simulink model "C_rho"  (R2020a)
settings: Solver=VariableStepAuto  StartTime=0.0  StopTime=10.0  RelTol=1e-3
settings Model: Creator=Willie  LastModifiedBy=Willie

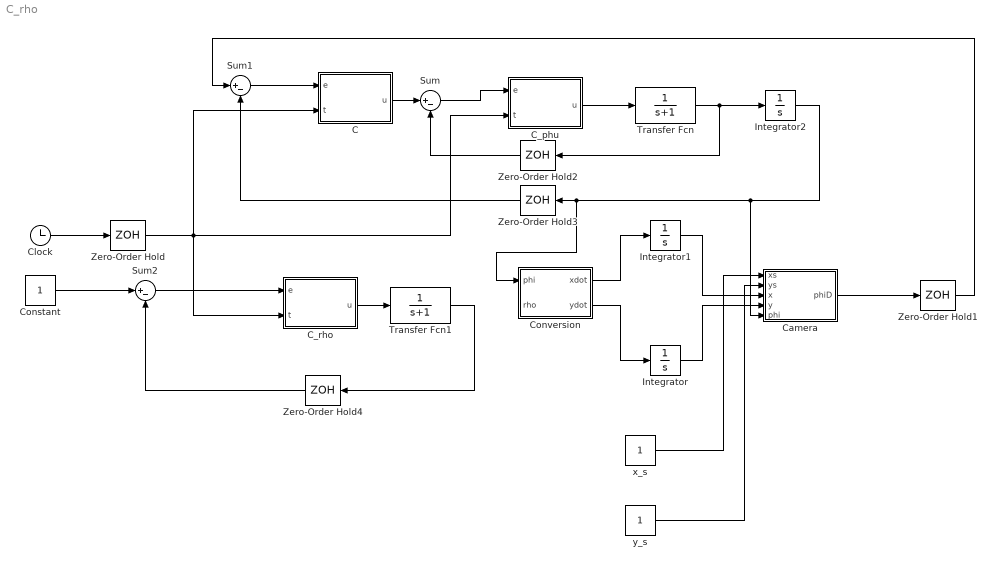
== system C_rho ==
  C : MATLAB Function  TreatAsAtomicUnit=on
  C_phu : MATLAB Function  TreatAsAtomicUnit=on
  C_rho : MATLAB Function  TreatAsAtomicUnit=on
  Camera : MATLAB Function  TreatAsAtomicUnit=on
  Clock : Clock
  Constant : Constant
  Conversion : MATLAB Function  TreatAsAtomicUnit=on
  Integrator : Integrator
  Integrator1 : Integrator
  Integrator2 : Integrator
  Sum : Sum  Inputs=|+-
  Sum1 : Sum  Inputs=|+-
  Sum2 : Sum  Inputs=|+-
  Transfer Fcn : TransferFcn  Denominator=[1 1]
  Transfer Fcn1 : TransferFcn  Denominator=[1 1]
  Zero-Order Hold{,1..4} (5 alike) : ZeroOrderHold  SampleTime=-1
  x_s : Constant
  y_s : Constant
  wires:
  Sum2/1 -> C_rho/1(e)
  Sum1/1 -> C/1(e)
  Clock/1 -> Zero-Order Hold/1
  Zero-Order Hold/1 -> C/2(t), C_phu/2(t), C_rho/2(t)
  C_rho/1(u) -> Transfer Fcn1/1
  Transfer Fcn1/1 -> Zero-Order Hold4/1
  Zero-Order Hold4/1 -> Sum2/2
  Constant/1 -> Sum2/1
  C/1(u) -> Sum/1
  Sum/1 -> C_phu/1(e)
  C_phu/1(u) -> Transfer Fcn/1
  Zero-Order Hold2/1 -> Sum/2
  Transfer Fcn/1 -> Integrator2/1, Zero-Order Hold2/1
  Integrator2/1 -> Camera/5(phi), Zero-Order Hold3/1, Conversion/1(phi)
  Zero-Order Hold3/1 -> Sum1/2
  Conversion/1(xdot) -> Integrator1/1
  Conversion/2(ydot) -> Integrator/1
  x_s/1 -> Camera/1(xs)
  y_s/1 -> Camera/2(ys)
  Integrator1/1 -> Camera/3(x)
  Integrator/1 -> Camera/4(y)
  Camera/1(phiD) -> Zero-Order Hold1/1
  Zero-Order Hold1/1 -> Sum1/1

== matlab function C_rho/C_phu ==
  data: e input; u output; t input
function u = fcn(e,t)

u = e;

== matlab function C_rho/Conversion ==
  data: xdot output; ydot output; phi input; rho input
function [xdot,ydot]= fcn(phi, rho)

y = u;

== matlab function C_rho/C ==
  data: e input; u output; t input
function u = fcn(e,t)

u = e*t;

== matlab function C_rho/C_rho ==
  data: e input; u output; t input
function u = fcn(e,t)

u = e;
u=t;

== matlab function C_rho/Camera ==
  data: xs input; phiD output; ys input; x input; y input; phi input
function phiD = fcn(xs,ys,x,y,phi)

y = u;
